simulink model "parte4_2"  (R2021b)
settings: Solver=FixedStepDiscrete  StartTime=0.0  StopTime=inf  FixedStep=.03  RelTol=1e-3  EnableMultiTasking=on
PostLoadFcn:
  | try,
  | codertarget.arduinobase.registry.setBaudRate(gcs,115200)
  | disp('baud rate set to 115200 for external mode hardware serial')
  | baudrate='set_to_115200'
  | catch
  | disp('baud rate setting not needed in this version')
  | end
undefined symbols (not defined in the file): DiscIntNeverNeededParam, EncCov, h, L1, Lcc, Ll
libraries: MinSegLibrary_M2V5 x2, simulink x1
settings Model: SimulationMode=external  ExtModeTrigDuration=2  Creator=Alec  LastModifiedBy=Dylan
settings SolverCC: AlgebraicLoopSolver=TrustRegion
settings DataIOCC: LimitDataPoints=on  SaveFormat=Array  ReturnWorkspaceOutputs=off
settings OptimizationCC: EnhancedBackFolding=on  PassReuseOutputArgsAs=Individual arguments  ExpressionDepthLimit=2147483647  ZeroExternalMemoryAtStartup=off  ZeroInternalMemoryAtStartup=off  MaxStackSize=64  OptimizeBlockOrder=speed  DifferentSizesBufferReuse=on  OptimizationCustomize=off  EfficientTunableParamExpr=on
settings DebuggingCC: UnderspecifiedInitializationDetection=Classic  MergeDetectMultiDrivingBlocksExec=none  ParameterTunabilityLossMsg=error  StateNameClashWarn=warning  SFUnexpectedBacktrackingDiag=warning  SFNoUnconditionalDefaultTransitionDiag=warning  SFExecutionAtInitializationDiag=none  SFMachineParentedDataDiag=warning  ArithmeticOperatorsInVariantConditions=warning
settings HardwareCC: ProdBitPerInt=16  ProdBitPerPointer=16  ProdBitPerSizeT=16  ProdBitPerPtrDiffT=16  ProdLargestAtomicFloat=None  ProdWordSize=8  ProdHWDeviceType=Atmel->AVR
settings ModelReferenceCC: PropagateSignalLabelsOutOfModel=off
settings SFSimCC: SimUseLocalCustomCode=off  MATLABDynamicMemAlloc=off  CustomCodeUndefinedFunction=UseInterfaceOnly
settings RTWCC: Description=Embedded Coder  SystemTargetFile=ert.tlc  HardwareBoard=Arduino Mega 2560  TemplateMakefile=ert_default_tmf  RTWVerbose=off  RTWUseLocalCustomCode=off  Toolchain=Arduino AVR  BuildConfiguration=Faster Runs
settings CodeAppCC: ForceParamTrailComments=on  IgnoreCustomStorageClasses=off  OperatorAnnotations=on  SimulinkDataObjDesc=on  SFDataObjDesc=on  CustomSymbolStrType=$N$R$M  InsertBlockDesc=on  InternalIdentifier=Classic
settings ERTTargetCC: SupportContinuousTime=on  SupportVariableSizeSignals=on  ExtModeTransport=3  ExtModeStaticAlloc=on  ExtModeStaticAllocSize=2048  ExtModeMexFile=ext_xcp  ExtModeIntrfLevel=Level2 - Open
settings ConfigComp: CovMetricSettings=dw  CovSaveCumulativeToWorkspaceVar=on  CovSaveSingleToWorkspaceVar=on  CovExternalEMLEnable=off

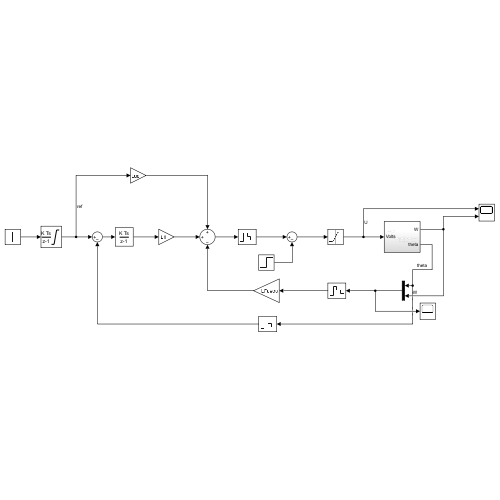
[thumbnail: Simulink's stored preview of the top-level diagram]
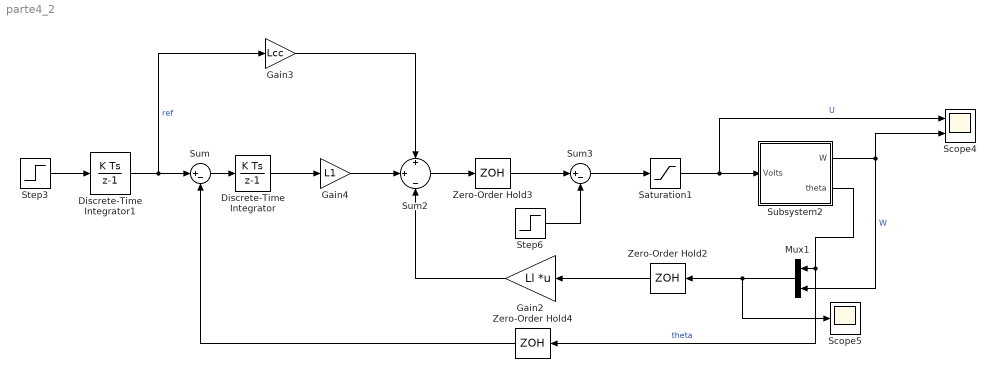
== system parte4_2 ==
  Discrete-Time Integrator : DiscreteIntegrator  SampleTime=h  ICPrevOutput=DiscIntNeverNeededParam  ICPrevScaledInput=DiscIntNeverNeededParam
  Discrete-Time Integrator1 : DiscreteIntegrator  SampleTime=h  LimitOutput=on  UpperSaturationLimit=70  LowerSaturationLimit=-70  ICPrevOutput=DiscIntNeverNeededParam  ICPrevScaledInput=DiscIntNeverNeededParam
  Gain2 : Gain  Gain=Ll  Multiplication=Matrix(K*u) (u vector)
  Gain3 : Gain  Gain=Lcc
  Gain4 : Gain  Gain=L1
  Mux1 : Mux  Inputs=2
  Saturation1 : Saturate  UpperLimit=4.8  LowerLimit=-4.8
  Scope4 : Scope  NumInputPorts=2
  Scope5 : Scope
  Step3 : Step  After=60  SampleTime=0
  Step6 : Step  Time=5  After=2  SampleTime=0
  Subsystem2 : Subsystem
  Sum : Sum  Inputs=|+-
  Sum2 : Sum  Inputs=+|+|-
  Sum3 : Sum  Inputs=|+-
  Zero-Order Hold2 : ZeroOrderHold  SampleTime=h
  Zero-Order Hold3 : ZeroOrderHold  SampleTime=h
  Zero-Order Hold4 : ZeroOrderHold  SampleTime=h
  wires:
  Zero-Order Hold4/1 -> Sum/2
  Gain4/1 -> Sum2/2
  Sum2/1 -> Zero-Order Hold3/1
  Discrete-Time Integrator/1 -> Gain4/1
  Sum/1 -> Discrete-Time Integrator/1
  Mux1/1 -> Scope5/1, Zero-Order Hold2/1
  Zero-Order Hold3/1 -> Sum3/1
  Saturation1/1 -> Subsystem2/1(Volts), Scope4/1  "U"
  Gain3/1 -> Sum2/1
  Subsystem2/1(W) -> Scope4/2, Mux1/2  "W"
  Gain2/1 -> Sum2/3
  Step6/1 -> Sum3/2
  Discrete-Time Integrator1/1 -> Sum/1, Gain3/1  "ref"
  Zero-Order Hold2/1 -> Gain2/1
  Sum3/1 -> Saturation1/1
  Subsystem2/2(theta) -> Zero-Order Hold4/1, Mux1/1  "theta"
  Step3/1 -> Discrete-Time Integrator1/1

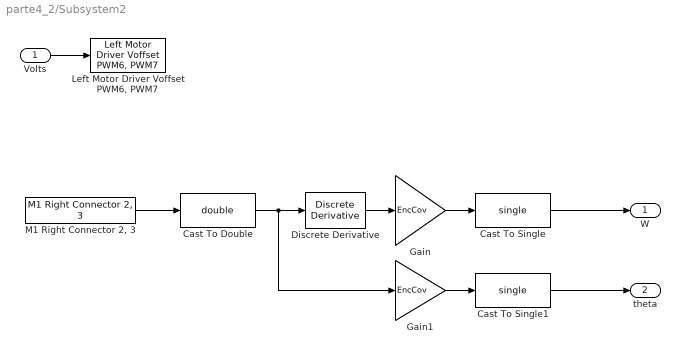
== system parte4_2/Subsystem2 ==
  Volts : Inport
  Cast To Double : DataTypeConversion  OutDataTypeStr=double
  Cast To Single : DataTypeConversion  OutDataTypeStr=single
  Cast To Single1 : DataTypeConversion  OutDataTypeStr=single
  Discrete Derivative : simulink/Discrete/Discrete Derivative  gainval=1.0  ICPrevScaledInput=0.0  OutMin=[]  OutMax=[]  OutDataType=fixdt(1, 16)  OutScaling=2^-10  DoSatur=off
  Gain : Gain  Gain=EncCov
  Gain1 : Gain  Gain=EncCov
  "Left Motor Driver Voffset PWM6, PWM7" : MinSegLibrary_M2V5/Left Motor Driver Voffset PWM6, PWM7  Vsupply=4.8  Voffset=0
      settings: SourceProductName=Rensselaer Arduino Support Package
  "M1 Right Connector 2, 3" : MinSegLibrary_M2V5/M1 Right Connector 2, 3  Encoder=0  PinA=2  PinB=3
      settings: SourceProductName=Rensselaer Arduino Support Package
  W : Outport
  theta : Outport  Port=2
  wires:
  Cast To Single/1 -> W/1
  Gain1/1 -> Cast To Single1/1
  Cast To Single1/1 -> theta/1
  "M1 Right Connector 2, 3"/1 -> Cast To Double/1
  Cast To Double/1 -> Gain1/1, Discrete Derivative/1
  Volts/1 -> "Left Motor Driver Voffset PWM6, PWM7"/1
  Discrete Derivative/1 -> Gain/1
  Gain/1 -> Cast To Single/1
